simulink library "EmptyInterpretation"  (R2022b)
settings: Solver=VariableStepAuto  StartTime=0.0  StopTime=10.0  RelTol=1e-3
settings Model: Creator=kl13806  LastModifiedBy=kl13806
settings SolverCC: AlgebraicLoopSolver=TrustRegion
settings DebuggingCC: UnconnectedInputMsg=warning  UnconnectedOutputMsg=warning  UnconnectedLineMsg=warning  SFMachineParentedDataDiag=warning  ArithmeticOperatorsInVariantConditions=warning
settings ModelReferenceCC: EnableRefExpFcnMdlSchedulingChecks=on
settings SFSimCC: SimUseLocalCustomCode=off  CustomCodeUndefinedFunction=UseInterfaceOnly
settings RTWCC: RTWUseLocalCustomCode=off  DLArmComputeVersion=19.05

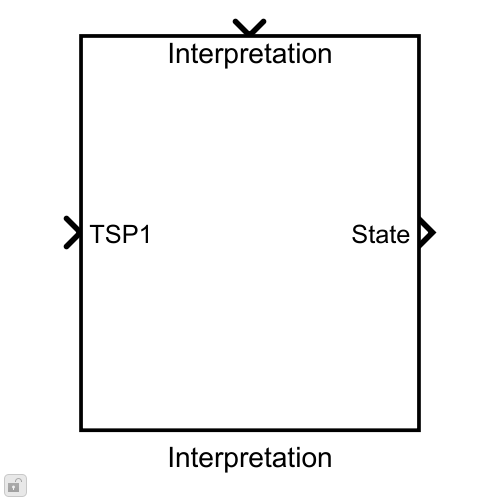
[thumbnail: Simulink's stored preview of the top-level diagram]
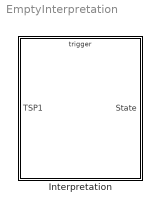
== system EmptyInterpretation ==
  Interpretation : MATLAB Function  TreatAsAtomicUnit=on  mask(Talaria Interpretation){}
      mask help: This MATLAB Function Block can be automatically inserted by several automation routines. Once placed, the block is ready to accept interpretation logic from the model designer.

== matlab function EmptyInterpretation/Interpretation ==
  data: State output; TSP1 input
  events: trigger input FUNCTION_CALL_EVENT
function State  = fcn(TSP1)
%#codegen

% Use one or more input Targe State Probes (TSP) or Captured State
% Constants to calculate an output state value that feeds into a StateVar
% block. Unlike tune translation code, this state interpretation code does
% not support variable size inputs - TSPs each have a fixed size. As a
% result, the input signals are just normal signal values that do *not*
% have .Value and .Size fields. No need for a custom bus!

% ----- To register an error, use the following method (works like printf):
%   InterpretError( <format string>, <arguments ... )
%   ... this error will cause the build process to abort.

% A trivial pass-through interpretation looks like this:
State = TSP1;
